simulink model "IK_iterative"  (R2018b)
settings: Solver=FixedStepAuto  StartTime=0.0  StopTime=TfMax  FixedStep=Ts  RelTol=1e-3
values from neighbouring files (symbols this model uses):
  JA = simplify(JA)    [getJacobA.m]
  q = symvar(Tq)    [getJacobA.m]    (also in getKinModel.m = sym('q',[1 n]))
undefined symbols (not defined in the file or in its folder): eStop, EulSim, JAMethod, K, q0, qd, subs, T04, xd
settings Model: Creator=adrimelu  LastModifiedBy=adrimelu

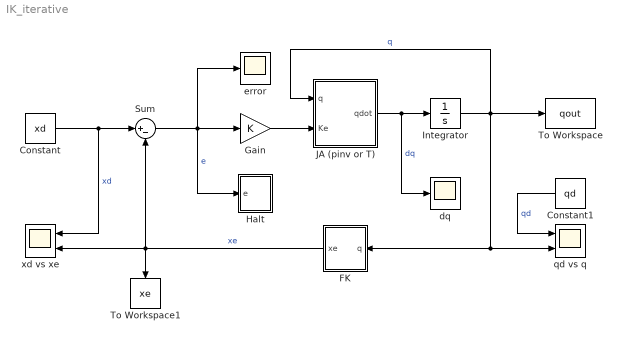
== system IK_iterative ==
  Constant : Constant  Value=xd
  Constant1 : Constant  Value=qd
  FK : Subsystem
  Gain : Gain  Gain=K
  Halt : Subsystem
  Integrator : Integrator  InitialCondition=q0
  JA (pinv or T) : Subsystem
  Sum : Sum  Inputs=|+-
  To Workspace : ToWorkspace  VariableName=qout  SaveFormat=Timeseries  SampleTime=-1
  To Workspace1 : ToWorkspace  VariableName=xe  SaveFormat=Timeseries  SampleTime=-1
  dq : Scope
  error : Scope
  qd vs q : Scope  NumInputPorts=2
  xd vs xe : Scope  NumInputPorts=2
  wires:
  JA (pinv or T)/1(qdot) -> dq/1, Integrator/1  "dq"
  Integrator/1 -> qd vs q/2, FK/1(q), To Workspace/1, JA (pinv or T)/1(q)  "q"
  Gain/1 -> JA (pinv or T)/2(Ke)
  FK/1(xe) -> To Workspace1/1, Sum/2, xd vs xe/2  "xe"
  Sum/1 -> Halt/1(e), error/1, Gain/1  "e"
  Constant/1 -> xd vs xe/1, Sum/1  "xd"
  Constant1/1 -> qd vs q/1  "qd"

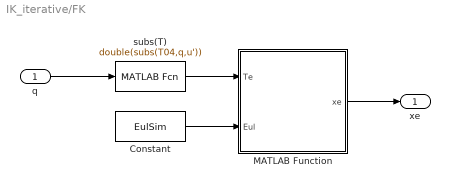
== system IK_iterative/FK ==
  q : Inport
  Constant : Constant  Value=EulSim
  MATLAB Function : MATLAB Function  TreatAsAtomicUnit=on
  subs(T) : MATLABFcn  MATLABFcn=double(subs(T04,q,u'))  OutputDimensions=[4 4]  Output1D=off
  xe : Outport
  wires:
  q/1 -> subs(T)/1
  MATLAB Function/1(xe) -> xe/1
  subs(T)/1 -> MATLAB Function/1(Te)
  Constant/1 -> MATLAB Function/2(Eul)

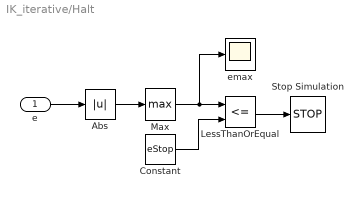
== system IK_iterative/Halt ==
  e : Inport
  Abs : Abs
  Constant : Constant  Value=eStop
  LessThanOrEqual : RelationalOperator  Operator=<=  OutDataTypeStr=boolean  RndMeth=Simplest
  Max : MinMax  Function=max
  Stop Simulation : Stop
  emax : Scope
  wires:
  e/1 -> Abs/1
  Constant/1 -> LessThanOrEqual/2
  Abs/1 -> Max/1
  LessThanOrEqual/1 -> Stop Simulation/1
  Max/1 -> emax/1, LessThanOrEqual/1

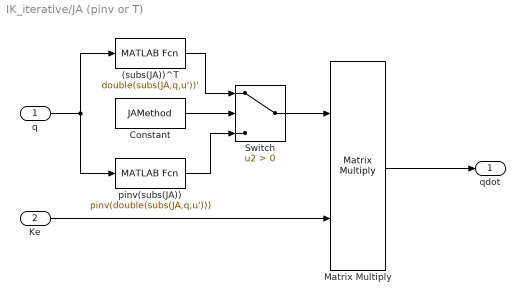
== system IK_iterative/JA (pinv or T) ==
  q : Inport
  Ke : Inport  Port=2
  (subs(JA))^T : MATLABFcn  MATLABFcn=double(subs(JA,q,u'))'  OutputDimensions=[4 6]  Output1D=off
  Constant : Constant  Value=JAMethod
  Matrix Multiply : Product  Multiplication=Matrix(*)
  Switch : Switch  Criteria=u2 > Threshold
  pinv(subs(JA)) : MATLABFcn  MATLABFcn=pinv(double(subs(JA,q,u')))  OutputDimensions=[4 6]  Output1D=off
  qdot : Outport
  wires:
  q/1 -> pinv(subs(JA))/1, (subs(JA))^T/1
  pinv(subs(JA))/1 -> Switch/3
  Ke/1 -> Matrix Multiply/2
  Matrix Multiply/1 -> qdot/1
  (subs(JA))^T/1 -> Switch/1
  Switch/1 -> Matrix Multiply/1
  Constant/1 -> Switch/2

== matlab function IK_iterative/FK/MATLAB Function ==
  data: Te input; xe output; Eul input
function xe = getxe(Te, Eul)
    
    pe = Te(1:3,4);
    phiz = atan2(Te(2,1), Te(1,1));
    
    if Eul == 0, phie = [0;0;phiz];
    elseif Eul == 1, phie = [phiz;pi;0];
    else, phie = [0;pi;-phiz];
    end

    xe = [pe; phie];
    
end
